simulink library "Lib_General"  (R2023a)
settings: Solver=VariableStepAuto  StartTime=0.0  StopTime=10.0  RelTol=1e-3
settings Model: Creator=62555  LastModifiedBy=62555

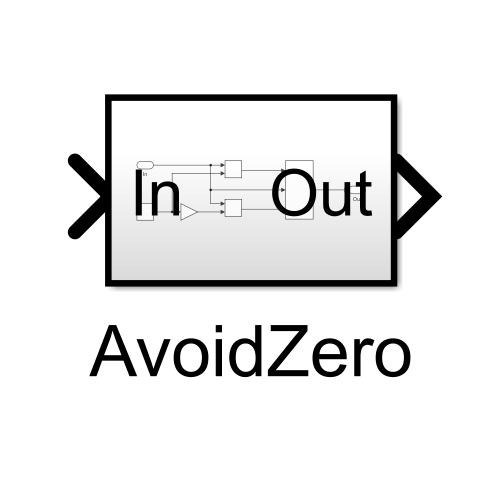
[thumbnail: Simulink's stored preview of the top-level diagram]
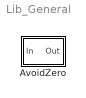
== system Lib_General ==
  AvoidZero : Subsystem  TreatAsAtomicUnit=on  RTWFileName=Lib_General
      settings: RTWFcnNameOpts=Use subsystem name  RTWFileNameOpts=User specified

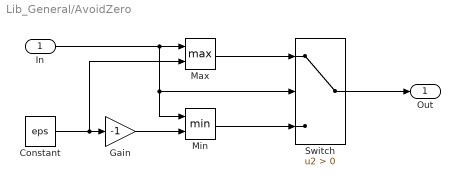
== system Lib_General/AvoidZero ==
  In : Inport
  Constant : Constant  Value=eps  OutDataTypeStr=single  SampleTime=-1
  Gain : Gain  Gain=-1
  Max : MinMax  Function=max  Inputs=2
  Min : MinMax  Inputs=2
  Switch : Switch  Criteria=u2 > Threshold  SaturateOnIntegerOverflow=off  InputSameDT=off
  Out : Outport
  wires:
  In/1 -> Min/1, Switch/2, Max/1
  Max/1 -> Switch/1
  Gain/1 -> Min/2
  Min/1 -> Switch/3
  Constant/1 -> Max/2, Gain/1
  Switch/1 -> Out/1
